simulink model "ProcNavNode"  (R2020a)
settings: Solver=FixedStepAuto  StartTime=0.0  StopTime=inf  FixedStep=1/60  RelTol=1e-3
model workspace (MAT data in the model file):
  SL_ROS_VariableLengthArrays_MaxSizes.CommonInfo.ArrayTruncateAction = 'EmitWarning'
  SL_ROS_VariableLengthArrays_MaxSizes.MsgTypeMap = containers.Map
  SL_ROS_VariableLengthArrays_MaxSizes.MsgTypeMap.serialization.keys = {}
  SL_ROS_VariableLengthArrays_MaxSizes.MsgTypeMap.serialization.values = {}
  SL_ROS_VariableLengthArrays_MaxSizes.MsgTypeMap.serialization.uniformity = 0
  SL_ROS_VariableLengthArrays_MaxSizes.MsgTypeMap.serialization.keyType = 'char'
  SL_ROS_VariableLengthArrays_MaxSizes.MsgTypeMap.serialization.valueType = 'any'
undefined symbols (not defined in the file): physics, simulation
libraries: robotlib x9, simulink_extras x1, simulink x1
settings Model: SimulationMode=external  PauseTimes=1000  Creator=Lamarre  LastModifiedBy=lamarre
settings OptimizationCC: EnhancedBackFolding=on  PassReuseOutputArgsAs=Individual arguments  ZeroExternalMemoryAtStartup=off  ZeroInternalMemoryAtStartup=off  MaxStackSize=64  OptimizeBlockOrder=speed  DifferentSizesBufferReuse=on  OptimizationCustomize=off  EfficientTunableParamExpr=on
settings DebuggingCC: ParameterTunabilityLossMsg=error  FcnCallInpInsideContextMsg=warning  UnderSpecifiedDimensionMsg=warning
settings HardwareCC: ProdBitPerPointer=32  ProdBitPerSizeT=32  ProdBitPerPtrDiffT=32  ProdLargestAtomicInteger=Long  ProdWordSize=32  ProdHWDeviceType=ARM Compatible->ARM 8
settings ModelReferenceCC: ModelReferenceNumInstancesAllowed=Single
settings SFSimCC: MATLABDynamicMemAlloc=off
settings RTWCC: SystemTargetFile=ert.tlc  HardwareBoard=Robot Operating System (ROS)  TemplateMakefile=ert_default_tmf  Toolchain=Catkin  BuildConfiguration=Faster Runs  TargetLang=C++
settings CodeAppCC: ForceParamTrailComments=on  IgnoreCustomStorageClasses=off  OperatorAnnotations=on  SimulinkDataObjDesc=on  SFDataObjDesc=on  InsertBlockDesc=on
settings ERTTargetCC: MultiInstanceERTCode=on  CodeInterfacePackaging=C++ class  SupportContinuousTime=on  RootIOFormat=Structure reference

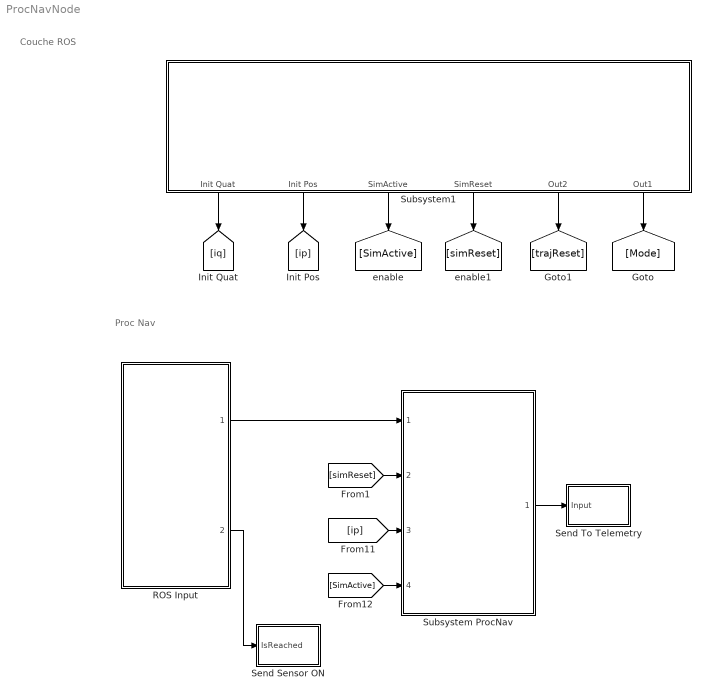
== system ProcNavNode ==
  note: Proc Nav
  note: Couche ROS
  ROS Input : Subsystem  ReferencedSubsystem=proc_nav_ros_input
  Send Sensor ON : Subsystem
  "Send To Telemetry " : Subsystem
  Subsystem ProcNav : Subsystem  ReferencedSubsystem=ProcNav
  Subsystem1 : Subsystem
      settings: PortSchema="{\"entries\":[{\"content\":{\"sides\":[{\"content\":{\"connectorIds\":[]},\"type\":\"ConnectorPlacement.EquallySpacedRectSide\",\"uuid\":\"274bdad9-d78d-43c8-9ae1-3ca28a37e384\"},{\"content\":{\"connectorIds\":[],\"side\":\"RIGHT\"},\"type\":\"ConnectorPlacement.EquallySpacedRectSide\",\"uuid\":\"7ee2482a-029c-4d86-ab0a-df49e4223d0b\"},{\"content\":{\"connectorIds\":[],\"side\":\"TOP\"},\"type\":\"ConnectorPlacement.EquallySpacedRectSide\",\"uuid\":\"c10c93c4-dac3-4bbe-8faf-09a38e374d51\"},{\"content\":{\"connectorIds\":[\"Out1\",\"Out2\",\"Out3\",\"Out4\",\"Out5\",\"Out6\"],\"side\":\"BOTTOM\"},\"type\":\"ConnectorPlacement.EquallySpacedRectSide\",\"uuid\":\"2cd10030-3eb5-48df-9d04-da9a86e3b973\"}]},\"type\":\"ConnectorPlacement.EquallySpacedConnector\",\"uuid\":\"6c3543f2-9cdd-4b68-a1ea-0df50348da33\"}],\"packageUris\":[\"http://schema.mathworks.com/mf0/Connector/19700101\"],\"version\":\"1.0\"}"
  wires:
  [SimActive] -> Subsystem ProcNav/4
  [simReset] -> Subsystem ProcNav/2
  ROS Input/1 -> Subsystem ProcNav/1
  ROS Input/2 -> Send Sensor ON/1(IsReached)
  Subsystem ProcNav/1 -> "Send To Telemetry "/1(Input)
  [ip] -> Subsystem ProcNav/3
  Subsystem1/1(Init Quat) -> [iq]
  Subsystem1/4(SimReset) -> [simReset]
  Subsystem1/3(SimActive) -> [SimActive]
  Subsystem1/5(Out2) -> [trajReset]
  Subsystem1/2(Init Pos) -> [ip]
  Subsystem1/6(Out1) -> [Mode]

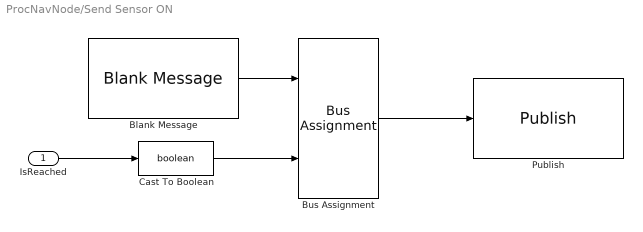
== system ProcNavNode/Send Sensor ON ==
  IsReached : Inport
  Blank Message : robotlib/Blank Message  messageClass=Message  entityType=std_msgs/Bool  messageType=std_msgs/Bool  SampleTime=inf
  Bus Assignment : BusAssignment  AssignedSignals=Data
  Cast To Boolean : DataTypeConversion  OutDataTypeStr=boolean
  Publish : robotlib/Publish  topicSource=Specify your own  topic=proc_control/sensor_on  messageType=std_msgs/Bool  messageQueueLength=1
  wires:
  Blank Message/1 -> Bus Assignment/1
  IsReached/1 -> Cast To Boolean/1
  Bus Assignment/1 -> Publish/1
  Cast To Boolean/1 -> Bus Assignment/2

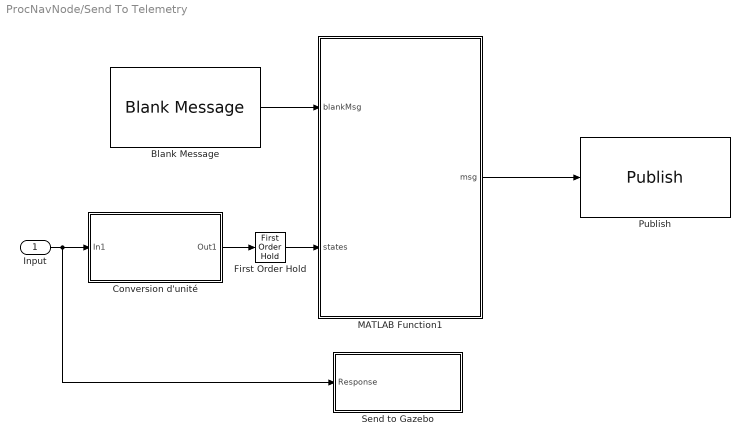
== system ProcNavNode/Send To Telemetry  ==
  Input : Inport
  Blank Message : robotlib/Blank Message  messageClass=Message  entityType=nav_msgs/Odometry  messageType=nav_msgs/Odometry  SampleTime=inf
  Conversion d'unité : Subsystem
  First Order Hold : FirstOrderHold  ErrorTolerance=inf  AllowContinuousInput=on
  MATLAB Function1 : MATLAB Function  TreatAsAtomicUnit=on  SystemSampleTime=1/30
  Publish : robotlib/Publish  topicSource=Specify your own  topic=/telemetry/auv_states/  messageType=nav_msgs/Odometry  messageQueueLength=1
  Send to Gazebo : Subsystem  InitFcn=""
  wires:
  Blank Message/1 -> MATLAB Function1/1(blankMsg)
  MATLAB Function1/1(msg) -> Publish/1
  Input/1 -> Send to Gazebo/1(Response), Conversion d'unité/1(In1)
  Conversion d'unité/1(Out1) -> First Order Hold/1
  First Order Hold/1 -> MATLAB Function1/2(states)

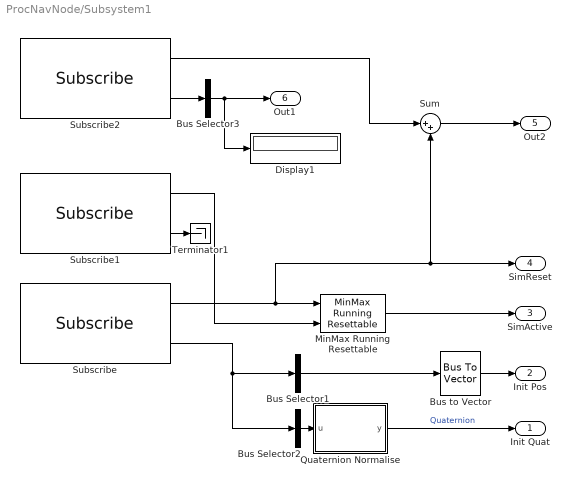
== system ProcNavNode/Subsystem1 ==
  Bus Selector1 : BusSelector  OutputSignals=Position.X,Position.Y,Position.Z  OutputAsBus=on
  Bus Selector2 : BusSelector  OutputSignals=Orientation.W,Orientation.Z,Orientation.Y,Orientation.X  OutputAsBus=on
  Bus Selector3 : BusSelector  OutputSignals=Data  OutputAsBus=on
  Bus to Vector : BusToVector
  Display1 : Display
  MinMax Running Resettable : simulink/Math Operations/MinMax Running Resettable  Function=max  vinit=0.0
  Quaternion Normalise : MATLAB Function  TreatAsAtomicUnit=on
  Subscribe : robotlib/Subscribe  topicSource=Select from ROS network  topic=/initial_condition  messageType=geometry_msgs/Pose  sampleTime=.25  messageQueueLength=1
  Subscribe1 : robotlib/Subscribe  topicSource=Specify your own  topic=/proc_control/kill  messageType=std_msgs/Bool  sampleTime=.25  messageQueueLength=1
  Subscribe2 : robotlib/Subscribe  topicSource=Specify your own  topic=/proc_control/set_mode  messageType=std_msgs/UInt8  sampleTime=.25  messageQueueLength=1
  Sum : Sum  Inputs=|++
  Terminator1 : Terminator
  Init Quat : Outport
  Init Pos : Outport  Port=2
  SimActive : Outport  Port=3
  SimReset : Outport  Port=4
  Out2 : Outport  Port=5
  Out1 : Outport  Port=6
  wires:
  Bus Selector2/1 -> Quaternion Normalise/1(u)
  Sum/1 -> Out2/1
  Bus Selector3/1 -> Display1/1, Out1/1
  Quaternion Normalise/1(y) -> Init Quat/1  "Quaternion"
  Subscribe/1 -> MinMax Running Resettable/1, Sum/2, SimReset/1
  Subscribe1/1 -> MinMax Running Resettable/2
  Subscribe1/2 -> Terminator1/1
  Bus Selector1/1 -> Bus to Vector/1
  Subscribe2/2 -> Bus Selector3/1
  Subscribe/2 -> Bus Selector2/1, Bus Selector1/1
  MinMax Running Resettable/1 -> SimActive/1
  Subscribe2/1 -> Sum/1
  Bus to Vector/1 -> Init Pos/1

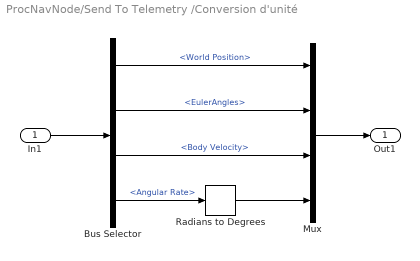
== system ProcNavNode/Send To Telemetry /Conversion d'unité ==
  In1 : Inport
  Bus Selector : BusSelector  OutputSignals=World Position,EulerAngles,Body Velocity,Angular Rate
  Mux : Mux
  Radians to Degrees : simulink_extras/Transformations/Radians to Degrees
  Out1 : Outport
  wires:
  Radians to Degrees/1 -> Mux/4
  Mux/1 -> Out1/1
  In1/1 -> Bus Selector/1
  Bus Selector/3 -> Mux/3  "<Body Velocity>"
  Bus Selector/2 -> Mux/2  "<EulerAngles>"
  Bus Selector/1 -> Mux/1  "<World Position>"
  Bus Selector/4 -> Radians to Degrees/1  "<Angular Rate>"

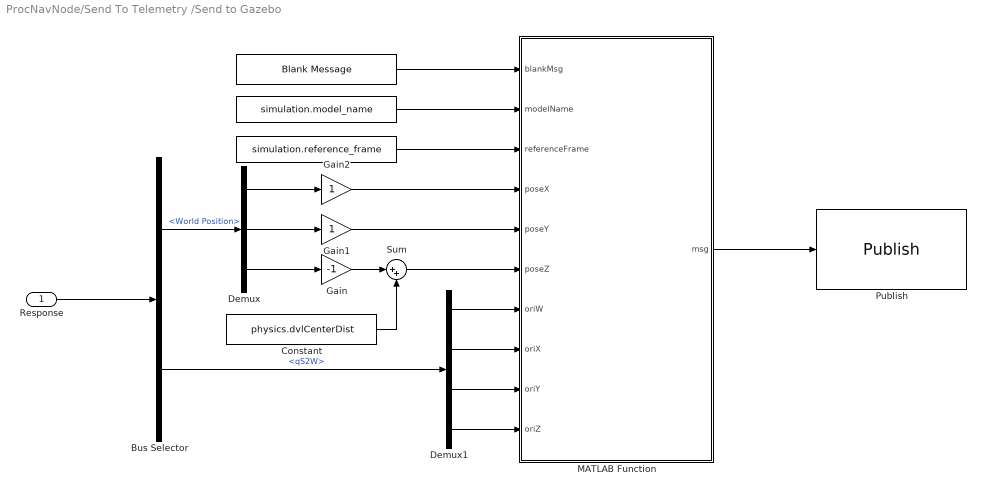
== system ProcNavNode/Send To Telemetry /Send to Gazebo ==
  Response : Inport
  " " : Constant  Value=simulation.model_name  VectorParams1D=off
  "  " : Constant  Value=simulation.reference_frame
  "   " : robotlib/Blank Message  messageClass=Message  entityType=gazebo_msgs/ModelState  messageType=gazebo_msgs/ModelState  SampleTime=1/60
  Bus Selector : BusSelector  OutputSignals=World Position,qS2W
  Constant : Constant  Value=physics.dvlCenterDist
  Demux : Demux  Outputs=3
  Demux1 : Demux
  Gain : Gain  Gain=-1
  Gain1 : Gain
  Gain2 : Gain
  MATLAB Function : MATLAB Function  TreatAsAtomicUnit=on  SystemSampleTime=1/60
  Publish : robotlib/Publish  topicSource=Select from ROS network  topic=/gazebo/set_model_state  messageType=gazebo_msgs/ModelState  messageQueueLength=1
      link override SinkBlock: ROSTopic=/gazebo/set_model_state  ROSMessageType=gazebo_msgs/ModelState  SLBusName=SL_Bus_plant_gazebo_msgs_ModelState  ModelName=plant  BlockId=Pub_plant_206
  Sum : Sum  Inputs=|++
  wires:
  Bus Selector/1 -> Demux/1  "<World Position>"
  Demux/1 -> Gain2/1
  Demux/2 -> Gain1/1
  Demux/3 -> Gain/1
  "   "/1 -> MATLAB Function/1(blankMsg)
  "  "/1 -> MATLAB Function/3(referenceFrame)
  " "/1 -> MATLAB Function/2(modelName)
  Gain1/1 -> MATLAB Function/5(poseY)
  Demux1/1 -> MATLAB Function/7(oriW)
  Demux1/2 -> MATLAB Function/8(oriX)
  Demux1/3 -> MATLAB Function/9(oriY)
  Demux1/4 -> MATLAB Function/10(oriZ)
  Gain2/1 -> MATLAB Function/4(poseX)
  MATLAB Function/1(msg) -> Publish/1
  Response/1 -> Bus Selector/1
  Gain/1 -> Sum/1
  Sum/1 -> MATLAB Function/6(poseZ)
  Constant/1 -> Sum/2
  Bus Selector/2 -> Demux1/1  "<qS2W>"

== matlab function ProcNavNode/Send To Telemetry /MATLAB Function1 ==
  data: blankMsg input; states input; msg output Bus: SL_Bus_ProcNavNode_nav_msgs_Odometry
function msg = SendOdometry(blankMsg, states)
msg = blankMsg;

% World Position 
    msg.Pose.Pose.Position.X = states(1);
    msg.Pose.Pose.Position.Y = states(2);
    msg.Pose.Pose.Position.Z = states(3);
    
% Sub atitude
    msg.Pose.Pose.Orientation.X = states(4);
    msg.Pose.Pose.Orientation.Y = states(5);
    msg.Pose.Pose.Orientation.Z = states(6);
    
% Body velocity
    msg.Twist.Twist.Linear.X = states(7);
    msg.Twist.Twist.Linear.Y = states(8);
    msg.Twist.Twist.Linear.Z = states(9);
    
% Angular rates
    msg.Twist.Twist.Angular.X = states(10);
    msg.Twist.Twist.Angular.Y = states(11);
    msg.Twist.Twist.Angular.Z = states(12);

== matlab function ProcNavNode/Subsystem1/Quaternion Normalise ==
  data: u input size=4; y output size=4
function y = Normalize(u)
%Normailse le quaternions pour éviter la distortions crée par l'erreur de
% de l'intégration.
d=norm(u);
n=u/d;
if isnan(n)
    y=[1;0;0;0];
else
    y = n;
end

== matlab function ProcNavNode/Send To Telemetry /Send to Gazebo/MATLAB Function ==
  data: blankMsg input; msg output Bus: SL_Bus_ProcNavNode_gazebo_msgs_ModelState; modelName input; referenceFrame input; poseX input; poseY input; poseZ input; oriW input; oriX input; oriY input; oriZ input
function msg = assignGazeboModelStateInput(blankMsg, modelName, referenceFrame, poseX, poseY, poseZ, oriW, oriX, oriY, oriZ)
% assignStringInput - Assign a string in a ROS message to specified input string
%
% MSG = assignStringInput(blankMsg, STR) assigns the input string, STR, to
%  a string field in the ROS message, blankMsg, and outputs the updated
%  ROS message.
%
%  Inputs
%    blankMsg: A bus for a 'std_msgs/String' message. This is 
%        used to initialize the output.
%    str: An array of uint8 that will be assigned to the 'Data' field
%        in blankMsg. The entire array is assumed to be a valid sequence of
%        character ASCII values.
% 
%  Outputs:
%    msg: A bus for a 'std_msgs/String' message, with the 'Data'
%        field set to a string.

%   Copyright 2015 The MathWorks, Inc.
%#codegen

% Note: The datatype of 'msg' has been explicitly set to the appropriate 
% Simulink bus type ("Bus: SL_Bus_robotROSMessageUsageExample_std_msgs_String"). 
%
% If the model name is changed, the datatype needs to be changed as well:
%   1) Click "Edit Data" in the Editor toolstrip to open "Ports and Data Manager"
%   2) Select "msg". From the "Type" dropdown, select "--- Refresh data types ---"
%   3) Set datatype to "Bus: SL_Bus_<modelname>_std_msgs_String"
   
msg = blankMsg;

strLength = length(modelName);
msg.ModelName(1:strLength) = modelName;
msg.ModelName_SL_Info.CurrentLength = uint32(strLength);

strLength = length(referenceFrame);
msg.ReferenceFrame(1:strLength) = referenceFrame;
msg.ReferenceFrame_SL_Info.CurrentLength = uint32(strLength);

msg.Pose.Position.X = poseX;
msg.Pose.Position.Y = poseY;
msg.Pose.Position.Z = poseZ;

msg.Pose.Orientation.X = oriX;
msg.Pose.Orientation.Y = oriY;
msg.Pose.Orientation.Z = oriZ;
msg.Pose.Orientation.W = oriW;
